simulink model "PSS2B_block"  (R2020a)
settings: Solver=FixedStepAuto  StartTime=0.0  StopTime=16.5  FixedStep=0.005  RelTol=1e-3
values from neighbouring files (symbols this model uses):
  K_S1 = 5    [PSS.m]    (also in PSS_parameter_change.m)
  K_S2 = 0.4    [PSS.m]    (also in PSS_parameter_change.m)
  K_S3 = 1    [PSS.m]    (also in PSS_parameter_change.m)
  T_1 = 0.2    [PSS.m]    (also in PSS_parameter_change.m)
  T_10 = 0.01    [PSS.m]    (also in PSS_parameter_change.m)
  T_11 = 0.01    [PSS.m]    (also in PSS_parameter_change.m)
  T_2 = 0.04    [PSS.m]    (also in PSS_parameter_change.m)
  T_3 = 0.36    [PSS.m]    (also in PSS_parameter_change.m)
  T_4 = 0.12    [PSS.m]    (also in PSS_parameter_change.m)
  T_6 = 0.02    [PSS.m]    (also in PSS_parameter_change.m = 0.01)
  T_7 = 2    [PSS.m]    (also in PSS_parameter_change.m)
  T_8 = 0.5    [PSS.m]    (also in PSS_parameter_change.m)
  T_9 = 0.1    [PSS.m]    (also in PSS_parameter_change.m)
  T_w1 = 4    [PSS.m]    (also in PSS_parameter_change.m = 2)
  T_w2 = 4    [PSS.m]    (also in PSS_parameter_change.m = 2)
  T_w3 = 2    [PSS.m]    (also in PSS_parameter_change.m)
  T_w4 = 2    [PSS.m]    (also in PSS_parameter_change.m)
  V_S1MAX = 0.8    [PSS.m]    (also in PSS_parameter_change.m)
  V_S1MIN = -0.8    [PSS.m]    (also in PSS_parameter_change.m)
  V_S2MAX = 1.25    [PSS.m]    (also in PSS_parameter_change.m)
  V_S2MIN = -1.25    [PSS.m]    (also in PSS_parameter_change.m)
  V_STMAX = 0.1    [PSS.m]    (also in PSS_parameter_change.m)
  V_STMIN = -0.1    [PSS.m]    (also in PSS_parameter_change.m)
settings Model: Creator=meagh  LastModifiedBy=meagh

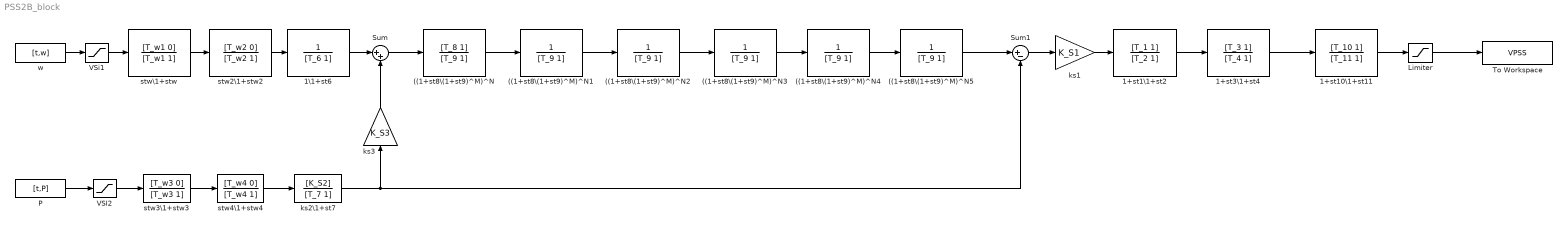
== system PSS2B_block ==
  ((1+st8\(1+st9)^M)^N : TransferFcn  Numerator=[T_8 1]  Denominator=[T_9 1]
  ((1+st8\(1+st9)^M)^N{1..5} (5 alike) : TransferFcn  Denominator=[T_9 1]
  1+st10\1+st11 : TransferFcn  Numerator=[T_10 1]  Denominator=[T_11 1]
  1+st1\1+st2 : TransferFcn  Numerator=[T_1 1]  Denominator=[T_2 1]
  1+st3\1+st4 : TransferFcn  Numerator=[T_3 1]  Denominator=[T_4 1]
  1\1+st6 : TransferFcn  Denominator=[T_6 1]
  "Limiter " : Saturate  UpperLimit=V_STMAX  LowerLimit=V_STMIN
  P : FromWorkspace  VariableName=[t,P]
  Sum : Sum  Inputs=|++
  Sum1 : Sum  Inputs=|+-
  To Workspace : ToWorkspace  VariableName=VPSS  SaveFormat=Timeseries  SampleTime=0.005
  VSI2 : Saturate  UpperLimit=V_S2MAX  LowerLimit=V_S2MIN
  VSi1 : Saturate  UpperLimit=V_S1MAX  LowerLimit=V_S1MIN
  ks1 : Gain  Gain=K_S1  SaturateOnIntegerOverflow=on  OutDataTypeStr=Inherit: Same as input  ParamDataTypeStr=Inherit: Same as input
  ks2\1+st7 : TransferFcn  Numerator=[K_S2]  Denominator=[T_7 1]
  ks3 : Gain  Gain=K_S3  SaturateOnIntegerOverflow=on  OutDataTypeStr=Inherit: Same as input  ParamDataTypeStr=Inherit: Same as input
  stw2\1+stw2 : TransferFcn  Numerator=[T_w2 0]  Denominator=[T_w2 1]
  stw3\1+stw3 : TransferFcn  Numerator=[T_w3 0]  Denominator=[T_w3 1]
  stw4\1+stw4 : TransferFcn  Numerator=[T_w4 0]  Denominator=[T_w4 1]
  stw\1+stw : TransferFcn  Numerator=[T_w1 0]  Denominator=[T_w1 1]
  w : FromWorkspace  VariableName=[t,w]
  wires:
  ks1/1 -> 1+st1\1+st2/1
  1+st3\1+st4/1 -> 1+st10\1+st11/1
  stw3\1+stw3/1 -> stw4\1+stw4/1
  ks2\1+st7/1 -> Sum1/2, ks3/1
  stw2\1+stw2/1 -> 1\1+st6/1
  ks3/1 -> Sum/2
  ((1+st8\(1+st9)^M)^N/1 -> ((1+st8\(1+st9)^M)^N1/1
  Sum1/1 -> ks1/1
  Sum/1 -> ((1+st8\(1+st9)^M)^N/1
  stw4\1+stw4/1 -> ks2\1+st7/1
  1\1+st6/1 -> Sum/1
  stw\1+stw/1 -> stw2\1+stw2/1
  1+st1\1+st2/1 -> 1+st3\1+st4/1
  P/1 -> VSI2/1
  VSI2/1 -> stw3\1+stw3/1
  VSi1/1 -> stw\1+stw/1
  w/1 -> VSi1/1
  1+st10\1+st11/1 -> "Limiter "/1
  "Limiter "/1 -> To Workspace/1
  ((1+st8\(1+st9)^M)^N1/1 -> ((1+st8\(1+st9)^M)^N2/1
  ((1+st8\(1+st9)^M)^N2/1 -> ((1+st8\(1+st9)^M)^N3/1
  ((1+st8\(1+st9)^M)^N3/1 -> ((1+st8\(1+st9)^M)^N4/1
  ((1+st8\(1+st9)^M)^N4/1 -> ((1+st8\(1+st9)^M)^N5/1
  ((1+st8\(1+st9)^M)^N5/1 -> Sum1/1
